simulink model "ap_12BAdapted"  (R2019b)
settings: Solver=FixedStepDiscrete  StartTime=0.0  StopTime=500  FixedStep=Ts  RelTol=1e-3  EnableMultiTasking=on
undefined symbols (not defined in the file): beaver_b, beaver_c, beaver_mass, beaver_S, Cl0, Cl_alpha2_dpt, Cl_beta, Cl_da, Cl_da_alpha, Cl_dr, Cl_p, Cl_r, Cm0, Cm_alpha, Cm_alpha2, Cm_beta2, Cm_de, Cm_df, Cm_dpt, Cm_q, Cm_r, Cn0, Cn_beta, Cn_beta3, Cn_da, Cn_dpt3, Cn_dr, Cn_p, Cn_q, Cn_r, Cx0, Cx_alpha, Cx_alpha2, Cx_alpha3, Cx_df, Cx_df_alpha, Cx_dpt, Cx_dpt2_alpha, Cx_dr, Cx_q, Cy0, Cy_beta, Cy_da, Cy_dr, Cy_dr_alpha, Cy_p, Cy_r, Cz0, Cz_alpha, Cz_alpha3, Cz_de, Cz_de_beta, Cz_df, Cz_df_alpha, Cz_dpt, Cz_q, d2r, fin_act_1, fin_act_2, fin_act_3 ... (+23)
libraries: simulink x10
(part 3 of 3)

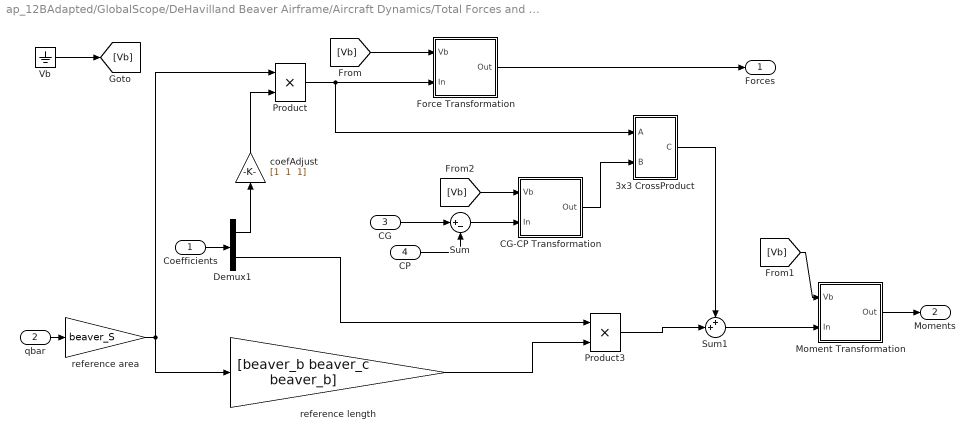
== system ap_12BAdapted/GlobalScope/DeHavilland Beaver Airframe/Aircraft Dynamics/Total Forces and Moments/Forces and Moments/Aero F&M ==
  Coefficients : Inport
  qbar : Inport  Port=2
  CG : Inport  Port=3
  CP : Inport  Port=4
  3x3 CrossProduct : Subsystem
  CG-CP Transformation : Subsystem  mask(Passive){}
      mask init:
      | %aeroicon('aeroblk');
  Demux1 : Demux  Outputs=[3,3]
  Force Transformation : Subsystem  mask(Passive){}
      mask init:
      | %aeroicon('aeroblk');
  Moment Transformation : Subsystem  mask(Passive){}
      mask init:
      | %aeroicon('aeroblk');
  Product : Product  SaturateOnIntegerOverflow=on  InputSameDT=on  OutDataTypeStr=Inherit: Same as first input
  Product3 : Product  SaturateOnIntegerOverflow=on  InputSameDT=on  OutDataTypeStr=Inherit: Same as first input
  Sum : Sum  Inputs=|+-  SaturateOnIntegerOverflow=on
  Sum1 : Sum  Inputs=++|  SaturateOnIntegerOverflow=on  InputSameDT=on  OutDataTypeStr=Inherit: Same as first input
  Vb : Ground
  coefAdjust : Gain  Gain="[1  1  1]"
  reference area : Gain  Gain=beaver_S  SaturateOnIntegerOverflow=on  OutDataTypeStr=Inherit: Same as input  ParamDataTypeStr=Inherit: Same as input
  reference length : Gain  Gain=[beaver_b beaver_c beaver_b]  SaturateOnIntegerOverflow=on  OutDataTypeStr=Inherit: Same as input  ParamDataTypeStr=Inherit: Same as input
  Forces : Outport  VectorParamsAs1DForOutWhenUnconnected=off
  Moments : Outport  Port=2  VectorParamsAs1DForOutWhenUnconnected=off
  wires:
  [Vb] -> Force Transformation/1(Vb)
  CP/1 -> Sum/2
  reference length/1 -> Product3/2
  Demux1/2 -> Product3/1
  qbar/1 -> reference area/1
  coefAdjust/1 -> Product/2
  Force Transformation/1(Out) -> Forces/1
  Demux1/1 -> coefAdjust/1
  Coefficients/1 -> Demux1/1
  [Vb] -> Moment Transformation/1(Vb)
  [Vb] -> CG-CP Transformation/1(Vb)
  CG-CP Transformation/1(Out) -> 3x3 CrossProduct/2(B)
  Product3/1 -> Sum1/2
  Vb/1 -> [Vb]
  reference area/1 -> reference length/1, Product/1
  Moment Transformation/1(Out) -> Moments/1
  Product/1 -> 3x3 CrossProduct/1(A), Force Transformation/2(In)
  Sum/1 -> CG-CP Transformation/2(In)
  Sum1/1 -> Moment Transformation/2(In)
  3x3 CrossProduct/1(C) -> Sum1/1
  CG/1 -> Sum/1

== system ap_12BAdapted/GlobalScope/DeHavilland Beaver Airframe/Aircraft Dynamics/6DoF (Quaternion)/Calculate DCM & Euler Angles/Quaternions to Direction Cosine Matrix/A11 ==
  normal(q) : Inport
  Demux : Demux
  Product{,1..3} (4 alike) : Product  RndMeth=Zero
  Sum : Sum  Inputs=++--
  A11 : Outport  VectorParamsAs1DForOutWhenUnconnected=off
  wires:
  Sum/1 -> A11/1
  Demux/4 -> Product/2, Product/1
  Demux/3 -> Product1/2, Product1/1
  Demux/2 -> Product2/2, Product2/1
  Demux/1 -> Product3/2, Product3/1
  Product3/1 -> Sum/1
  Product2/1 -> Sum/2
  Product1/1 -> Sum/3
  Product/1 -> Sum/4
  normal(q)/1 -> Demux/1

== system ap_12BAdapted/GlobalScope/DeHavilland Beaver Airframe/Aircraft Dynamics/6DoF (Quaternion)/Calculate DCM & Euler Angles/Quaternions to Direction Cosine Matrix/A12 ==
  normal(q) : Inport
  Demux : Demux
  Gain : Gain  Gain=2
  Product2 : Product  RndMeth=Zero
  Product3 : Product  RndMeth=Zero
  Sum : Sum  Inputs=|++
  A12 : Outport  VectorParamsAs1DForOutWhenUnconnected=off
  wires:
  Product2/1 -> Sum/2
  Product3/1 -> Sum/1
  Sum/1 -> Gain/1
  Demux/1 -> Product3/2
  Demux/2 -> Product2/1
  Demux/4 -> Product3/1
  Demux/3 -> Product2/2
  normal(q)/1 -> Demux/1
  Gain/1 -> A12/1

== system ap_12BAdapted/GlobalScope/DeHavilland Beaver Airframe/Aircraft Dynamics/6DoF (Quaternion)/Calculate DCM & Euler Angles/Quaternions to Direction Cosine Matrix/A13 ==
  normal(q) : Inport
  Demux : Demux
  Gain : Gain  Gain=2
  Product1 : Product  RndMeth=Zero
  Product2 : Product  RndMeth=Zero
  Sum : Sum  Inputs=|-+
  A13 : Outport  VectorParamsAs1DForOutWhenUnconnected=off
  wires:
  Demux/1 -> Product1/1
  Product1/1 -> Sum/1
  Product2/1 -> Sum/2
  Demux/4 -> Product2/2
  Demux/2 -> Product2/1
  Demux/3 -> Product1/2
  normal(q)/1 -> Demux/1
  Gain/1 -> A13/1
  Sum/1 -> Gain/1

== system ap_12BAdapted/GlobalScope/DeHavilland Beaver Airframe/Aircraft Dynamics/6DoF (Quaternion)/Calculate DCM & Euler Angles/Quaternions to Direction Cosine Matrix/A21 ==
  normal(q) : Inport
  Demux : Demux
  Gain : Gain  Gain=2
  Product2 : Product  RndMeth=Zero
  Product3 : Product  RndMeth=Zero
  Sum : Sum  Inputs=|-+
  A21 : Outport  VectorParamsAs1DForOutWhenUnconnected=off
  wires:
  Gain/1 -> A21/1
  normal(q)/1 -> Demux/1
  Demux/3 -> Product2/2
  Demux/4 -> Product3/1
  Demux/2 -> Product2/1
  Demux/1 -> Product3/2
  Sum/1 -> Gain/1
  Product3/1 -> Sum/1
  Product2/1 -> Sum/2

== system ap_12BAdapted/GlobalScope/DeHavilland Beaver Airframe/Aircraft Dynamics/6DoF (Quaternion)/Calculate DCM & Euler Angles/Quaternions to Direction Cosine Matrix/A22 ==
  normal(q) : Inport
  Demux : Demux
  Product{,1..3} (4 alike) : Product  RndMeth=Zero
  Sum : Sum  Inputs=+-+-
  A22 : Outport  VectorParamsAs1DForOutWhenUnconnected=off
  wires:
  normal(q)/1 -> Demux/1
  Product/1 -> Sum/4
  Product1/1 -> Sum/3
  Product2/1 -> Sum/2
  Product3/1 -> Sum/1
  Demux/1 -> Product3/1, Product3/2
  Demux/2 -> Product2/1, Product2/2
  Demux/3 -> Product1/1, Product1/2
  Demux/4 -> Product/1, Product/2
  Sum/1 -> A22/1

== system ap_12BAdapted/GlobalScope/DeHavilland Beaver Airframe/Aircraft Dynamics/6DoF (Quaternion)/Calculate DCM & Euler Angles/Quaternions to Direction Cosine Matrix/A23 ==
  normal(q) : Inport
  Demux : Demux
  Gain : Gain  Gain=2
  Product1 : Product  RndMeth=Zero
  Product2 : Product  RndMeth=Zero
  Sum : Sum  Inputs=|++
  A23 : Outport  VectorParamsAs1DForOutWhenUnconnected=off
  wires:
  Demux/4 -> Product2/2
  Product2/1 -> Sum/2
  Product1/1 -> Sum/1
  Sum/1 -> Gain/1
  Demux/1 -> Product1/1
  Demux/2 -> Product1/2
  Demux/3 -> Product2/1
  Gain/1 -> A23/1
  normal(q)/1 -> Demux/1

== system ap_12BAdapted/GlobalScope/DeHavilland Beaver Airframe/Aircraft Dynamics/6DoF (Quaternion)/Calculate DCM & Euler Angles/Quaternions to Direction Cosine Matrix/A31 ==
  normal(q) : Inport
  Demux : Demux
  Gain : Gain  Gain=2
  Product1 : Product  RndMeth=Zero
  Product2 : Product  RndMeth=Zero
  Sum : Sum  Inputs=|++
  A31 : Outport  VectorParamsAs1DForOutWhenUnconnected=off
  wires:
  Sum/1 -> Gain/1
  Gain/1 -> A31/1
  normal(q)/1 -> Demux/1
  Demux/3 -> Product1/2
  Demux/2 -> Product2/1
  Demux/4 -> Product2/2
  Product2/1 -> Sum/2
  Product1/1 -> Sum/1
  Demux/1 -> Product1/1

== system ap_12BAdapted/GlobalScope/DeHavilland Beaver Airframe/Aircraft Dynamics/6DoF (Quaternion)/Calculate DCM & Euler Angles/Quaternions to Direction Cosine Matrix/A32 ==
  normal(q) : Inport
  Demux : Demux
  Gain : Gain  Gain=2
  Product1 : Product  RndMeth=Zero
  Product2 : Product  RndMeth=Zero
  Sum : Sum  Inputs=|-+
  A32 : Outport  VectorParamsAs1DForOutWhenUnconnected=off
  wires:
  normal(q)/1 -> Demux/1
  Gain/1 -> A32/1
  Demux/3 -> Product2/1
  Demux/2 -> Product1/2
  Demux/1 -> Product1/1
  Sum/1 -> Gain/1
  Product1/1 -> Sum/1
  Product2/1 -> Sum/2
  Demux/4 -> Product2/2

== system ap_12BAdapted/GlobalScope/DeHavilland Beaver Airframe/Aircraft Dynamics/6DoF (Quaternion)/Calculate DCM & Euler Angles/Quaternions to Direction Cosine Matrix/A33 ==
  normal(q) : Inport
  Demux : Demux
  Product{,1..3} (4 alike) : Product  RndMeth=Zero
  Sum : Sum  Inputs=+--+
  A33 : Outport  VectorParamsAs1DForOutWhenUnconnected=off
  wires:
  normal(q)/1 -> Demux/1
  Product/1 -> Sum/4
  Product1/1 -> Sum/3
  Product2/1 -> Sum/2
  Product3/1 -> Sum/1
  Demux/1 -> Product3/1, Product3/2
  Demux/2 -> Product2/1, Product2/2
  Demux/3 -> Product1/1, Product1/2
  Demux/4 -> Product/1, Product/2
  Sum/1 -> A33/1

== system ap_12BAdapted/GlobalScope/DeHavilland Beaver Airframe/Aircraft Dynamics/6DoF (Quaternion)/Calculate DCM & Euler Angles/Quaternions to Direction Cosine Matrix/Create 3x3 Matrix ==
  M11 : Inport  PortDimensions=1
  M12 : Inport  Port=2  PortDimensions=1
  M13 : Inport  Port=3  PortDimensions=1
  M21 : Inport  Port=4  PortDimensions=1
  M22 : Inport  Port=5  PortDimensions=1
  M23 : Inport  Port=6  PortDimensions=1
  M31 : Inport  Port=7  PortDimensions=1
  M32 : Inport  Port=8  PortDimensions=1
  M33 : Inport  Port=9  PortDimensions=1
  Reshape (9) to [3x3] column-major : Reshape  OutputDimensionality=Customize  OutputDimensions=[3,3]
  Vector Concatenate : Concatenate  NumInputs=9
  Matrix : Outport  PortDimensions=[3 3]  VectorParamsAs1DForOutWhenUnconnected=off
  wires:
  M33/1 -> Vector Concatenate/9
  M23/1 -> Vector Concatenate/8
  M13/1 -> Vector Concatenate/7
  M32/1 -> Vector Concatenate/6
  Reshape (9) to [3x3] column-major/1 -> Matrix/1
  M22/1 -> Vector Concatenate/5
  M12/1 -> Vector Concatenate/4
  M31/1 -> Vector Concatenate/3
  M21/1 -> Vector Concatenate/2
  M11/1 -> Vector Concatenate/1
  Vector Concatenate/1 -> Reshape (9) to [3x3] column-major/1

== system ap_12BAdapted/GlobalScope/DeHavilland Beaver Airframe/Aircraft Dynamics/6DoF (Quaternion)/Calculate DCM & Euler Angles/Quaternions to Direction Cosine Matrix/Quaternion Normalize ==
  q : Inport  Unit=1
  Demux : Demux
  Mux : Mux
  Product{,1..3} (4 alike) : Product  Inputs=*/
  Quaternion Modulus : Subsystem  mask(Quaternion Modulus){}
      mask help: shared_aeroblks:sharedaeroblkutil:blockQuaternionModulusDesc
      mask init:
      | if license('test','aerospace_blockset')
      |     aerosharedicon('shared');
      | elseif license('test','powertrain_blockset')
      |     sharedautoicon('shared');
      | end
      mask Help: eval('if license(''test'',''aerospace_blockset'')aerosharedhelp;elseif license(''test'',''powertrain_blockset'')sharedautohelp;end')
  normal(q) : Outport  Unit=1  VectorParamsAs1DForOutWhenUnconnected=off
  wires:
  Product3/1 -> Mux/4
  Product2/1 -> Mux/3
  Product1/1 -> Mux/2
  Product/1 -> Mux/1
  Quaternion Modulus/1(|q|) -> Product3/2, Product2/2, Product/2, Product1/2
  q/1 -> Demux/1, Quaternion Modulus/1(q)
  Mux/1 -> normal(q)/1
  Demux/1 -> Product/1
  Demux/2 -> Product1/1
  Demux/3 -> Product2/1
  Demux/4 -> Product3/1

== system ap_12BAdapted/GlobalScope/DeHavilland Beaver Airframe/Aircraft Dynamics/6DoF (Quaternion)/Calculate DCM & Euler Angles/Quaternions to Rotation Angles (ZYX)/Quaternion Normalize ==
  q : Inport
  Demux : Demux
  Mux : Mux
  Product{,1..3} (4 alike) : Product  Inputs=*/
  Quaternion Modulus : Subsystem
  normal(q) : Outport  VectorParamsAs1DForOutWhenUnconnected=off
  wires:
  Product3/1 -> Mux/4
  Product1/1 -> Mux/2
  Demux/1 -> Product/1
  Quaternion Modulus/1(|q|) -> Product1/2, Product/2, Product2/2, Product3/2
  Mux/1 -> normal(q)/1
  q/1 -> Quaternion Modulus/1(q), Demux/1
  Product/1 -> Mux/1
  Demux/3 -> Product2/1
  Demux/4 -> Product3/1
  Product2/1 -> Mux/3
  Demux/2 -> Product1/1

== system ap_12BAdapted/GlobalScope/DeHavilland Beaver Airframe/Aircraft Dynamics/6DoF (Quaternion)/Calculate omega_dot/3x3 CrossProduct/Subsystem ==
  A : Inport
  B : Inport  Port=2
  Demux : Demux  Outputs=3
  Demux1 : Demux  Outputs=3
  Mux : Mux  Inputs=3
  i x j : Product  SaturateOnIntegerOverflow=on  InputSameDT=on  OutDataTypeStr=Inherit: Same as first input
  j x k : Product  SaturateOnIntegerOverflow=on  InputSameDT=on  OutDataTypeStr=Inherit: Same as first input
  k x i : Product  SaturateOnIntegerOverflow=on  InputSameDT=on  OutDataTypeStr=Inherit: Same as first input
  Out1 : Outport  VectorParamsAs1DForOutWhenUnconnected=off
  wires:
  Demux1/3 -> j x k/2
  Demux/2 -> j x k/1
  Demux/3 -> k x i/1
  Demux1/1 -> k x i/2
  Demux1/2 -> i x j/2
  Demux/1 -> i x j/1
  i x j/1 -> Mux/3
  k x i/1 -> Mux/2
  j x k/1 -> Mux/1
  B/1 -> Demux1/1
  A/1 -> Demux/1
  Mux/1 -> Out1/1

== system ap_12BAdapted/GlobalScope/DeHavilland Beaver Airframe/Aircraft Dynamics/6DoF (Quaternion)/Calculate omega_dot/3x3 CrossProduct/Subsystem1 ==
  A : Inport
  B : Inport  Port=2
  Demux : Demux  Outputs=3
  Demux1 : Demux  Outputs=3
  Mux : Mux  Inputs=3
  i x k : Product  SaturateOnIntegerOverflow=on  InputSameDT=on  OutDataTypeStr=Inherit: Same as first input
  j x i : Product  SaturateOnIntegerOverflow=on  InputSameDT=on  OutDataTypeStr=Inherit: Same as first input
  k x j : Product  SaturateOnIntegerOverflow=on  InputSameDT=on  OutDataTypeStr=Inherit: Same as first input
  Out1 : Outport  VectorParamsAs1DForOutWhenUnconnected=off
  wires:
  j x i/1 -> Mux/3
  i x k/1 -> Mux/2
  k x j/1 -> Mux/1
  Mux/1 -> Out1/1
  Demux1/1 -> j x i/2
  Demux/2 -> j x i/1
  Demux1/3 -> i x k/2
  Demux/1 -> i x k/1
  Demux1/2 -> k x j/2
  Demux/3 -> k x j/1
  B/1 -> Demux1/1
  A/1 -> Demux/1

== system ap_12BAdapted/GlobalScope/DeHavilland Beaver Airframe/Aircraft Dynamics/Total Forces and Moments/Actuators/sof/ResetIntegratorInternal ==
  note: ic
  note: Level Reset Integration With Saturation
      | y(n) = y(n-1) + K*Ts*u(n-1)
  U : Inport
  R : Inport  Port=2
  ic : Inport  Port=3
  Constant : Constant  Value=1.0
  Constant1 : Constant  Value=Ts
  Product : Product  RndMeth=Zero
  Product1 : Product  RndMeth=Zero
  Sum3 : Sum
  Switch : Switch  Criteria=u2 ~= 0
  Switch1 : Switch  Criteria=u2 ~= 0
  X : UnitDelay  SampleTime=Ts  HasFrameUpgradeWarning=on
  Y : Outport  VectorParamsAs1DForOutWhenUnconnected=off
  wires:
  Product1/1 -> Sum3/1
  U/1 -> Product1/2
  Sum3/1 -> Switch1/3
  Product/1 -> Product1/1
  ic/1 -> Switch1/1, Switch/1
  Constant1/1 -> Product/2  "deltaT"
  Switch1/1 -> X/1
  Constant/1 -> Product/1  "gain"
  Switch/1 -> Y/1, Sum3/2
  R/1 -> Switch1/2, Switch/2
  X/1 -> Switch/3

== system ap_12BAdapted/GlobalScope/DeHavilland Beaver Airframe/Aircraft Dynamics/Total Forces and Moments/Actuators/sof/ResetIntegratorInternal1 ==
  note: Level Reset Integration With Saturation
      | y(n) = y(n-1) + K*Ts*u(n-1)
  note: ic
  U : Inport
  R : Inport  Port=2
  ic : Inport  Port=3
  Constant : Constant  Value=1.0
  Constant1 : Constant  Value=Ts
  Product : Product  RndMeth=Zero
  Product1 : Product  RndMeth=Zero
  Saturation : Saturate  UpperLimit=fin_max  LowerLimit=fin_min
  Sum3 : Sum
  Switch : Switch  Criteria=u2 ~= 0
  Switch1 : Switch  Criteria=u2 ~= 0
  X : UnitDelay  SampleTime=Ts  HasFrameUpgradeWarning=on
  Y : Outport  VectorParamsAs1DForOutWhenUnconnected=off
  wires:
  X/1 -> Switch/3
  R/1 -> Switch/2, Switch1/2
  Saturation/1 -> Sum3/2, Y/1
  Constant/1 -> Product/1  "gain"
  Switch1/1 -> X/1
  Constant1/1 -> Product/2  "deltaT"
  ic/1 -> Switch/1, Switch1/1
  Switch/1 -> Saturation/1
  Product/1 -> Product1/1
  Sum3/1 -> Switch1/3
  U/1 -> Product1/2
  Product1/1 -> Sum3/1

== system ap_12BAdapted/GlobalScope/DeHavilland Beaver Airframe/Aircraft Dynamics/Total Forces and Moments/Actuators/sof/ic1 ==
  Constant : Constant  Value=0
  Constant1 : Constant  Value=fin_act_1
  Unit Delay : UnitDelay  InitialCondition=1  SampleTime=-1  HasFrameUpgradeWarning=on
  R : Outport  VectorParamsAs1DForOutWhenUnconnected=off
  IC : Outport  Port=2  VectorParamsAs1DForOutWhenUnconnected=off
  wires:
  Constant1/1 -> IC/1
  Unit Delay/1 -> R/1
  Constant/1 -> Unit Delay/1

== system ap_12BAdapted/GlobalScope/DeHavilland Beaver Airframe/Aircraft Dynamics/Total Forces and Moments/Actuators/sof/ic3 ==
  Constant : Constant  Value=0
  Constant1 : Constant  Value=0.0
  Unit Delay : UnitDelay  InitialCondition=1  SampleTime=-1  HasFrameUpgradeWarning=on
  R : Outport  VectorParamsAs1DForOutWhenUnconnected=off
  IC : Outport  Port=2  VectorParamsAs1DForOutWhenUnconnected=off
  wires:
  Constant/1 -> Unit Delay/1
  Unit Delay/1 -> R/1
  Constant1/1 -> IC/1

== system ap_12BAdapted/GlobalScope/DeHavilland Beaver Airframe/Aircraft Dynamics/Total Forces and Moments/Actuators/sof1/ResetIntegratorInternal ==
  note: Level Reset Integration With Saturation
      | y(n) = y(n-1) + K*Ts*u(n-1)
  note: ic
  U : Inport
  R : Inport  Port=2
  ic : Inport  Port=3
  Constant : Constant  Value=1.0
  Constant1 : Constant  Value=Ts
  Product : Product  RndMeth=Zero
  Product1 : Product  RndMeth=Zero
  Sum3 : Sum
  Switch : Switch  Criteria=u2 ~= 0
  Switch1 : Switch  Criteria=u2 ~= 0
  X : UnitDelay  SampleTime=Ts  HasFrameUpgradeWarning=on
  Y : Outport  VectorParamsAs1DForOutWhenUnconnected=off
  wires:
  X/1 -> Switch/3
  R/1 -> Switch/2, Switch1/2
  Switch/1 -> Sum3/2, Y/1
  Constant/1 -> Product/1  "gain"
  Switch1/1 -> X/1
  Constant1/1 -> Product/2  "deltaT"
  ic/1 -> Switch/1, Switch1/1
  Product/1 -> Product1/1
  Sum3/1 -> Switch1/3
  U/1 -> Product1/2
  Product1/1 -> Sum3/1

== system ap_12BAdapted/GlobalScope/DeHavilland Beaver Airframe/Aircraft Dynamics/Total Forces and Moments/Actuators/sof1/ResetIntegratorInternal1 ==
  note: ic
  note: Level Reset Integration With Saturation
      | y(n) = y(n-1) + K*Ts*u(n-1)
  U : Inport
  R : Inport  Port=2
  ic : Inport  Port=3
  Constant : Constant  Value=1.0
  Constant1 : Constant  Value=Ts
  Product : Product  RndMeth=Zero
  Product1 : Product  RndMeth=Zero
  Saturation : Saturate  UpperLimit=fin_max  LowerLimit=fin_min
  Sum3 : Sum
  Switch : Switch  Criteria=u2 ~= 0
  Switch1 : Switch  Criteria=u2 ~= 0
  X : UnitDelay  SampleTime=Ts  HasFrameUpgradeWarning=on
  Y : Outport  VectorParamsAs1DForOutWhenUnconnected=off
  wires:
  Product1/1 -> Sum3/1
  U/1 -> Product1/2
  Sum3/1 -> Switch1/3
  Product/1 -> Product1/1
  Switch/1 -> Saturation/1
  ic/1 -> Switch1/1, Switch/1
  Constant1/1 -> Product/2  "deltaT"
  Switch1/1 -> X/1
  Constant/1 -> Product/1  "gain"
  Saturation/1 -> Y/1, Sum3/2
  R/1 -> Switch1/2, Switch/2
  X/1 -> Switch/3

== system ap_12BAdapted/GlobalScope/DeHavilland Beaver Airframe/Aircraft Dynamics/Total Forces and Moments/Actuators/sof1/ic1 ==
  Constant : Constant  Value=0
  Constant1 : Constant  Value=fin_act_2
  Unit Delay : UnitDelay  InitialCondition=1  SampleTime=-1  HasFrameUpgradeWarning=on
  R : Outport  VectorParamsAs1DForOutWhenUnconnected=off
  IC : Outport  Port=2  VectorParamsAs1DForOutWhenUnconnected=off
  wires:
  Constant/1 -> Unit Delay/1
  Unit Delay/1 -> R/1
  Constant1/1 -> IC/1

== system ap_12BAdapted/GlobalScope/DeHavilland Beaver Airframe/Aircraft Dynamics/Total Forces and Moments/Actuators/sof1/ic3 ==
  Constant : Constant  Value=0
  Constant1 : Constant  Value=0.0
  Unit Delay : UnitDelay  InitialCondition=1  SampleTime=-1  HasFrameUpgradeWarning=on
  R : Outport  VectorParamsAs1DForOutWhenUnconnected=off
  IC : Outport  Port=2  VectorParamsAs1DForOutWhenUnconnected=off
  wires:
  Constant1/1 -> IC/1
  Unit Delay/1 -> R/1
  Constant/1 -> Unit Delay/1

== system ap_12BAdapted/GlobalScope/DeHavilland Beaver Airframe/Aircraft Dynamics/Total Forces and Moments/Actuators/sof2/ResetIntegratorInternal ==
  note: ic
  note: Level Reset Integration With Saturation
      | y(n) = y(n-1) + K*Ts*u(n-1)
  U : Inport
  R : Inport  Port=2
  ic : Inport  Port=3
  Constant : Constant  Value=1.0
  Constant1 : Constant  Value=Ts
  Product : Product  RndMeth=Zero
  Product1 : Product  RndMeth=Zero
  Sum3 : Sum
  Switch : Switch  Criteria=u2 ~= 0
  Switch1 : Switch  Criteria=u2 ~= 0
  X : UnitDelay  SampleTime=Ts  HasFrameUpgradeWarning=on
  Y : Outport  VectorParamsAs1DForOutWhenUnconnected=off
  wires:
  Product1/1 -> Sum3/1
  U/1 -> Product1/2
  Sum3/1 -> Switch1/3
  Product/1 -> Product1/1
  ic/1 -> Switch1/1, Switch/1
  Constant1/1 -> Product/2  "deltaT"
  Switch1/1 -> X/1
  Constant/1 -> Product/1  "gain"
  Switch/1 -> Y/1, Sum3/2
  R/1 -> Switch1/2, Switch/2
  X/1 -> Switch/3

== system ap_12BAdapted/GlobalScope/DeHavilland Beaver Airframe/Aircraft Dynamics/Total Forces and Moments/Actuators/sof2/ResetIntegratorInternal1 ==
  note: Level Reset Integration With Saturation
      | y(n) = y(n-1) + K*Ts*u(n-1)
  note: ic
  U : Inport
  R : Inport  Port=2
  ic : Inport  Port=3
  Constant : Constant  Value=1.0
  Constant1 : Constant  Value=Ts
  Product : Product  RndMeth=Zero
  Product1 : Product  RndMeth=Zero
  Saturation : Saturate  UpperLimit=fin_max  LowerLimit=fin_min
  Sum3 : Sum
  Switch : Switch  Criteria=u2 ~= 0
  Switch1 : Switch  Criteria=u2 ~= 0
  X : UnitDelay  SampleTime=Ts  HasFrameUpgradeWarning=on
  Y : Outport  VectorParamsAs1DForOutWhenUnconnected=off
  wires:
  X/1 -> Switch/3
  R/1 -> Switch/2, Switch1/2
  Saturation/1 -> Sum3/2, Y/1
  Constant/1 -> Product/1  "gain"
  Switch1/1 -> X/1
  Constant1/1 -> Product/2  "deltaT"
  ic/1 -> Switch/1, Switch1/1
  Switch/1 -> Saturation/1
  Product/1 -> Product1/1
  Sum3/1 -> Switch1/3
  U/1 -> Product1/2
  Product1/1 -> Sum3/1

== system ap_12BAdapted/GlobalScope/DeHavilland Beaver Airframe/Aircraft Dynamics/Total Forces and Moments/Actuators/sof2/ic1 ==
  Constant : Constant  Value=0
  Constant1 : Constant  Value=fin_act_3
  Unit Delay : UnitDelay  InitialCondition=1  SampleTime=-1  HasFrameUpgradeWarning=on
  R : Outport  VectorParamsAs1DForOutWhenUnconnected=off
  IC : Outport  Port=2  VectorParamsAs1DForOutWhenUnconnected=off
  wires:
  Constant1/1 -> IC/1
  Unit Delay/1 -> R/1
  Constant/1 -> Unit Delay/1

== system ap_12BAdapted/GlobalScope/DeHavilland Beaver Airframe/Aircraft Dynamics/Total Forces and Moments/Actuators/sof2/ic3 ==
  Constant : Constant  Value=0
  Constant1 : Constant  Value=0.0
  Unit Delay : UnitDelay  InitialCondition=1  SampleTime=-1  HasFrameUpgradeWarning=on
  R : Outport  VectorParamsAs1DForOutWhenUnconnected=off
  IC : Outport  Port=2  VectorParamsAs1DForOutWhenUnconnected=off
  wires:
  Constant/1 -> Unit Delay/1
  Unit Delay/1 -> R/1
  Constant1/1 -> IC/1

== system ap_12BAdapted/GlobalScope/DeHavilland Beaver Airframe/Aircraft Dynamics/Total Forces and Moments/Aerodynamics/Actuator Increments/Aileron ==
  alpha : Inport
  Actuators : Inport  Port=2
  Gain1 : Gain  Gain=0  SaturateOnIntegerOverflow=on  OutDataTypeStr=Inherit: Same as input  ParamDataTypeStr=Inherit: Same as input
  Gain2 : Gain  Gain=Cy_da  SaturateOnIntegerOverflow=on  OutDataTypeStr=Inherit: Same as input  ParamDataTypeStr=Inherit: Same as input
  Gain3 : Gain  Gain=0  SaturateOnIntegerOverflow=on  OutDataTypeStr=Inherit: Same as input  ParamDataTypeStr=Inherit: Same as input
  Gain4 : Gain  Gain=Cn_da  SaturateOnIntegerOverflow=on  OutDataTypeStr=Inherit: Same as input  ParamDataTypeStr=Inherit: Same as input
  Gain5 : Gain  Gain=0  SaturateOnIntegerOverflow=on  OutDataTypeStr=Inherit: Same as input  ParamDataTypeStr=Inherit: Same as input
  Gain6 : Gain  Gain=Cl_da  SaturateOnIntegerOverflow=on  OutDataTypeStr=Inherit: Same as input  ParamDataTypeStr=Inherit: Same as input
  Gain7 : Gain  Gain=Cl_da_alpha  SaturateOnIntegerOverflow=on  OutDataTypeStr=Inherit: Same as input  ParamDataTypeStr=Inherit: Same as input
  Mux1 : Mux  Inputs=6
  Product4 : Product  SaturateOnIntegerOverflow=on  InputSameDT=on  OutDataTypeStr=Inherit: Same as first input
  Selector1 : Selector  InputPortWidth=4  IndexOptions=Index vector (dialog)  Indices=2  OutputSizes=1
  Sum1 : Sum  Inputs=++|  SaturateOnIntegerOverflow=on
  delCoeff : Outport  VectorParamsAs1DForOutWhenUnconnected=off
  wires:
  Gain6/1 -> Sum1/1
  Sum1/1 -> Mux1/4
  Gain7/1 -> Sum1/2
  Product4/1 -> Gain7/1
  Gain1/1 -> Mux1/1  "Cx"
  alpha/1 -> Product4/2
  Actuators/1 -> Selector1/1
  Mux1/1 -> delCoeff/1
  Gain2/1 -> Mux1/2  "Cy"
  Gain3/1 -> Mux1/3  "Cz"
  Gain5/1 -> Mux1/5  "Cm"
  Gain4/1 -> Mux1/6
  Selector1/1 -> Gain1/1, Gain2/1, Gain3/1, Gain6/1, Product4/1, Gain5/1, Gain4/1

== system ap_12BAdapted/GlobalScope/DeHavilland Beaver Airframe/Aircraft Dynamics/Total Forces and Moments/Aerodynamics/Actuator Increments/Elevator ==
  Actuators : Inport
  Beta : Inport  Port=2
  Constant1 : Constant  Value=0
  Gain1 : Gain  Gain=Cz_de  SaturateOnIntegerOverflow=on  OutDataTypeStr=Inherit: Same as input  ParamDataTypeStr=Inherit: Same as input
  Gain2 : Gain  Gain=Cz_de_beta  SaturateOnIntegerOverflow=on  OutDataTypeStr=Inherit: Same as input  ParamDataTypeStr=Inherit: Same as input
  Gain3 : Gain  Gain=Cm_de  SaturateOnIntegerOverflow=on  OutDataTypeStr=Inherit: Same as input  ParamDataTypeStr=Inherit: Same as input
  Mux1 : Mux  Inputs=6
  Product1 : Product  SaturateOnIntegerOverflow=on  InputSameDT=on  OutDataTypeStr=Inherit: Same as first input
  Product2 : Product  SaturateOnIntegerOverflow=on  InputSameDT=on  OutDataTypeStr=Inherit: Same as first input
  Selector1 : Selector  InputPortWidth=4  IndexOptions=Index vector (dialog)  Indices=1  OutputSizes=1
  Sum1 : Sum  SaturateOnIntegerOverflow=on
  delCoeff : Outport  VectorParamsAs1DForOutWhenUnconnected=off
  wires:
  Gain3/1 -> Mux1/5
  Gain1/1 -> Sum1/2
  Gain2/1 -> Sum1/1
  Sum1/1 -> Mux1/3
  Product2/1 -> Gain2/1
  Beta/1 -> Product1/2, Product1/1
  Mux1/1 -> delCoeff/1
  Selector1/1 -> Gain3/1, Product2/2, Gain1/1
  Constant1/1 -> Mux1/1, Mux1/2, Mux1/4, Mux1/6
  Actuators/1 -> Selector1/1
  Product1/1 -> Product2/1

== system ap_12BAdapted/GlobalScope/DeHavilland Beaver Airframe/Aircraft Dynamics/Total Forces and Moments/Aerodynamics/Actuator Increments/Flap ==
  Alpha : Inport
  Actuators : Inport  Port=2
  Constant1 : Constant  Value=0
  Constant2 : Constant  Value=0
  Constant3 : Constant  Value=0
  Gain1 : Gain  Gain=Cx_df  SaturateOnIntegerOverflow=on  OutDataTypeStr=Inherit: Same as input  ParamDataTypeStr=Inherit: Same as input
  Gain2 : Gain  Gain=Cx_df_alpha  SaturateOnIntegerOverflow=on  OutDataTypeStr=Inherit: Same as input  ParamDataTypeStr=Inherit: Same as input
  Gain3 : Gain  Gain=Cz_df  SaturateOnIntegerOverflow=on  OutDataTypeStr=Inherit: Same as input  ParamDataTypeStr=Inherit: Same as input
  Gain4 : Gain  Gain=Cz_df_alpha  SaturateOnIntegerOverflow=on  OutDataTypeStr=Inherit: Same as input  ParamDataTypeStr=Inherit: Same as input
  Gain5 : Gain  Gain=Cm_df  SaturateOnIntegerOverflow=on  OutDataTypeStr=Inherit: Same as input  ParamDataTypeStr=Inherit: Same as input
  Mux1 : Mux  Inputs=6
  Product1 : Product  SaturateOnIntegerOverflow=on  InputSameDT=on  OutDataTypeStr=Inherit: Same as first input
  Product4 : Product  SaturateOnIntegerOverflow=on  InputSameDT=on  OutDataTypeStr=Inherit: Same as first input
  Selector1 : Selector  InputPortWidth=4  IndexOptions=Index vector (dialog)  Indices=4  OutputSizes=1
  Sum1 : Sum  SaturateOnIntegerOverflow=on
  Sum2 : Sum  SaturateOnIntegerOverflow=on
  delCoeff : Outport  VectorParamsAs1DForOutWhenUnconnected=off
  wires:
  Selector1/1 -> Gain1/1, Product4/1, Product1/1, Gain3/1, Gain5/1
  Actuators/1 -> Selector1/1
  Gain5/1 -> Mux1/5
  Gain3/1 -> Sum2/1
  Gain4/1 -> Sum2/2
  Product1/1 -> Gain4/1
  Gain1/1 -> Sum1/1
  Gain2/1 -> Sum1/2
  Product4/1 -> Gain2/1
  Alpha/1 -> Product1/2, Product4/2
  Mux1/1 -> delCoeff/1
  Sum1/1 -> Mux1/1
  Sum2/1 -> Mux1/3
  Constant1/1 -> Mux1/2
  Constant2/1 -> Mux1/4
  Constant3/1 -> Mux1/6

== system ap_12BAdapted/GlobalScope/DeHavilland Beaver Airframe/Aircraft Dynamics/Total Forces and Moments/Aerodynamics/Actuator Increments/Rudder ==
  Alpha : Inport
  Actuators : Inport  Port=2
  Constant1 : Constant  Value=0
  Constant2 : Constant  Value=0
  Gain1 : Gain  Gain=Cl_dr  SaturateOnIntegerOverflow=on  OutDataTypeStr=Inherit: Same as input  ParamDataTypeStr=Inherit: Same as input
  Gain2 : Gain  Gain=Cn_dr  SaturateOnIntegerOverflow=on  OutDataTypeStr=Inherit: Same as input  ParamDataTypeStr=Inherit: Same as input
  Gain3 : Gain  Gain=Cy_dr_alpha  SaturateOnIntegerOverflow=on  OutDataTypeStr=Inherit: Same as input  ParamDataTypeStr=Inherit: Same as input
  Gain4 : Gain  Gain=Cy_dr  SaturateOnIntegerOverflow=on  OutDataTypeStr=Inherit: Same as input  ParamDataTypeStr=Inherit: Same as input
  Gain5 : Gain  Gain=Cx_dr  SaturateOnIntegerOverflow=on  OutDataTypeStr=Inherit: Same as input  ParamDataTypeStr=Inherit: Same as input
  Mux1 : Mux  Inputs=6
  Product1 : Product  SaturateOnIntegerOverflow=on  InputSameDT=on  OutDataTypeStr=Inherit: Same as first input
  Selector1 : Selector  InputPortWidth=4  IndexOptions=Index vector (dialog)  Indices=3  OutputSizes=1
  Sum1 : Sum  SaturateOnIntegerOverflow=on
  delCoeff : Outport  VectorParamsAs1DForOutWhenUnconnected=off
  wires:
  Gain5/1 -> Mux1/1
  Gain4/1 -> Sum1/1
  Gain3/1 -> Sum1/2
  Gain1/1 -> Mux1/4
  Gain2/1 -> Mux1/6
  Product1/1 -> Gain3/1
  Alpha/1 -> Product1/2
  Mux1/1 -> delCoeff/1
  Actuators/1 -> Selector1/1
  Sum1/1 -> Mux1/2
  Constant1/1 -> Mux1/3
  Constant2/1 -> Mux1/5
  Selector1/1 -> Gain5/1, Gain4/1, Product1/1, Gain1/1, Gain2/1

== system ap_12BAdapted/GlobalScope/DeHavilland Beaver Airframe/Aircraft Dynamics/Total Forces and Moments/Aerodynamics/Body Rate Damping/p ==
  Constant1 : Constant  Value=0
  Constant2 : Constant  Value=Cy_p
  Constant3 : Constant  Value=Cl_p
  Constant4 : Constant  Value=Cn_p
  Mux1 : Mux  Inputs=6
  delCoeff : Outport  VectorParamsAs1DForOutWhenUnconnected=off
  wires:
  Constant2/1 -> Mux1/2
  Mux1/1 -> delCoeff/1
  Constant1/1 -> Mux1/5, Mux1/3, Mux1/1
  Constant4/1 -> Mux1/6
  Constant3/1 -> Mux1/4

== system ap_12BAdapted/GlobalScope/DeHavilland Beaver Airframe/Aircraft Dynamics/Total Forces and Moments/Aerodynamics/Body Rate Damping/q ==
  Constant1 : Constant  Value=0
  Constant2 : Constant  Value=Cz_q
  Constant3 : Constant  Value=Cx_q
  Constant4 : Constant  Value=Cm_q
  Constant5 : Constant  Value=Cn_q
  Mux1 : Mux  Inputs=6
  delCoeff : Outport  VectorParamsAs1DForOutWhenUnconnected=off
  wires:
  Constant2/1 -> Mux1/3
  Constant5/1 -> Mux1/6
  Constant1/1 -> Mux1/4, Mux1/2
  Constant4/1 -> Mux1/5
  Constant3/1 -> Mux1/1
  Mux1/1 -> delCoeff/1

== system ap_12BAdapted/GlobalScope/DeHavilland Beaver Airframe/Aircraft Dynamics/Total Forces and Moments/Aerodynamics/Body Rate Damping/r ==
  Constant : Constant  Value=0
  Constant1 : Constant  Value=Cy_r
  Constant2 : Constant  Value=Cl_r
  Constant3 : Constant  Value=Cm_r
  Constant4 : Constant  Value=Cn_r
  Mux1 : Mux  Inputs=6
  delCoeff : Outport  VectorParamsAs1DForOutWhenUnconnected=off
  wires:
  Constant3/1 -> Mux1/5
  Constant1/1 -> Mux1/2
  Constant4/1 -> Mux1/6
  Constant2/1 -> Mux1/4
  Constant/1 -> Mux1/3, Mux1/1
  Mux1/1 -> delCoeff/1

== system ap_12BAdapted/GlobalScope/DeHavilland Beaver Airframe/Aircraft Dynamics/Total Forces and Moments/Engine /pow/calc ==
  In1 : Inport
  Constant4 : Constant  Value=408.0
  Constant5 : Constant  Value=1.0
  Demux : Demux  Outputs=3
  Gain2 : Gain  Gain=0.0965  SaturateOnIntegerOverflow=on  OutDataTypeStr=Inherit: Same as input  ParamDataTypeStr=Inherit: Same as input
  Gain4 : Gain  Gain=0.8163  SaturateOnIntegerOverflow=on  OutDataTypeStr=Inherit: Same as input  ParamDataTypeStr=Inherit: Same as input
  Product2 : Product  RndMeth=Zero
  Sum1 : Sum  Inputs=+-|  SaturateOnIntegerOverflow=on
  Sum2 : Sum  Inputs=+-|  SaturateOnIntegerOverflow=on
  Terminator : Terminator
  Out1 : Outport  VectorParamsAs1DForOutWhenUnconnected=off
  wires:
  In1/1 -> Demux/1
  Product2/1 -> Out1/1
  Sum2/1 -> Product2/2
  Constant5/1 -> Sum2/1
  Gain4/1 -> Sum2/2
  Constant4/1 -> Sum1/1
  Demux/1 -> Gain2/1
  Demux/2 -> Terminator/1
  Gain2/1 -> Sum1/2
  Sum1/1 -> Product2/1
  Demux/3 -> Gain4/1

== system ap_12BAdapted/GlobalScope/DeHavilland Beaver Airframe/Aircraft Dynamics/Total Forces and Moments/Engine /pow/calc1 ==
  In1 : Inport
  Constant1 : Constant  Value=2010
  Constant2 : Constant  Value=7.4
  Demux : Demux  Outputs=2
  Product1 : Product  RndMeth=Zero
  Sum3 : Sum  Inputs=++|  SaturateOnIntegerOverflow=on
  Sum4 : Sum  Inputs=|++  SaturateOnIntegerOverflow=on
  Out1 : Outport  VectorParamsAs1DForOutWhenUnconnected=off
  wires:
  In1/1 -> Demux/1
  Demux/1 -> Sum3/2
  Constant1/1 -> Sum3/1
  Sum3/1 -> Product1/1
  Demux/2 -> Sum4/1
  Constant2/1 -> Sum4/2
  Sum4/1 -> Product1/2
  Product1/1 -> Out1/1

== system ap_12BAdapted/GlobalScope/DeHavilland Beaver Airframe/Aircraft Dynamics/Total Forces and Moments/Forces and Moments/Aero F&M/3x3 CrossProduct ==
  A : Inport
  B : Inport  Port=2
  "A " : InportShadow
  "B " : InportShadow  Port=2
  Subsystem : Subsystem
  Subsystem1 : Subsystem
  Sum : Sum  Inputs=+|-  SaturateOnIntegerOverflow=on  InputSameDT=on  OutDataTypeStr=Inherit: Same as first input
  C : Outport  VectorParamsAs1DForOutWhenUnconnected=off
  wires:
  "A "/1 -> Subsystem1/1(A)
  Subsystem/1(Out1) -> Sum/1
  B/1 -> Subsystem/2(B)
  Sum/1 -> C/1
  "B "/1 -> Subsystem1/2(B)
  Subsystem1/1(Out1) -> Sum/2
  A/1 -> Subsystem/1(A)

== system ap_12BAdapted/GlobalScope/DeHavilland Beaver Airframe/Aircraft Dynamics/Total Forces and Moments/Forces and Moments/Aero F&M/CG-CP Transformation ==
  Vb : Inport
  In : Inport  Port=2
  Terminator1 : Terminator
  Out : Outport  VectorParamsAs1DForOutWhenUnconnected=off
  wires:
  In/1 -> Out/1
  Vb/1 -> Terminator1/1

== system ap_12BAdapted/GlobalScope/DeHavilland Beaver Airframe/Aircraft Dynamics/Total Forces and Moments/Forces and Moments/Aero F&M/Force Transformation ==
  Vb : Inport
  In : Inport  Port=2
  Terminator1 : Terminator
  Out : Outport  VectorParamsAs1DForOutWhenUnconnected=off
  wires:
  In/1 -> Out/1
  Vb/1 -> Terminator1/1

== system ap_12BAdapted/GlobalScope/DeHavilland Beaver Airframe/Aircraft Dynamics/Total Forces and Moments/Forces and Moments/Aero F&M/Moment Transformation ==
  Vb : Inport
  In : Inport  Port=2
  Terminator1 : Terminator
  Out : Outport  VectorParamsAs1DForOutWhenUnconnected=off
  wires:
  In/1 -> Out/1
  Vb/1 -> Terminator1/1

== system ap_12BAdapted/GlobalScope/DeHavilland Beaver Airframe/Aircraft Dynamics/6DoF (Quaternion)/Calculate DCM & Euler Angles/Quaternions to Direction Cosine Matrix/Quaternion Normalize/Quaternion Modulus ==
  q : Inport  Unit=1
  Quaternion Norm : Subsystem  mask(Quaternion Norm){}
      mask help: shared_aeroblks:sharedaeroblkutil:blockQuaternionNormDesc
      mask init:
      | if license('test','aerospace_blockset')
      |     aerosharedicon('shared');
      | elseif license('test','powertrain_blockset')
      |     sharedautoicon('shared');
      | end
      mask Help: eval('if license(''test'',''aerospace_blockset'')aerosharedhelp;elseif license(''test'',''powertrain_blockset'')sharedautohelp;end')
  sqrt : Sqrt  AlgorithmType=Newton-Raphson  SaturateOnIntegerOverflow=on
  |q| : Outport  Unit=1  VectorParamsAs1DForOutWhenUnconnected=off
  wires:
  Quaternion Norm/1(norm(q)) -> sqrt/1
  q/1 -> Quaternion Norm/1(q)
  sqrt/1 -> |q|/1

== system ap_12BAdapted/GlobalScope/DeHavilland Beaver Airframe/Aircraft Dynamics/6DoF (Quaternion)/Calculate DCM & Euler Angles/Quaternions to Rotation Angles (ZYX)/Quaternion Normalize/Quaternion Modulus ==
  q : Inport
  Quaternion Norm : Subsystem
  sqrt : Sqrt  AlgorithmType=Newton-Raphson  SaturateOnIntegerOverflow=on
  |q| : Outport  VectorParamsAs1DForOutWhenUnconnected=off
  wires:
  Quaternion Norm/1(norm(q)) -> sqrt/1
  sqrt/1 -> |q|/1
  q/1 -> Quaternion Norm/1(q)

== system ap_12BAdapted/GlobalScope/DeHavilland Beaver Airframe/Aircraft Dynamics/Total Forces and Moments/Forces and Moments/Aero F&M/3x3 CrossProduct/Subsystem ==
  A : Inport
  B : Inport  Port=2
  Demux : Demux  Outputs=3
  Demux1 : Demux  Outputs=3
  Mux : Mux  Inputs=3
  i x j : Product  SaturateOnIntegerOverflow=on  InputSameDT=on  OutDataTypeStr=Inherit: Same as first input
  j x k : Product  SaturateOnIntegerOverflow=on  InputSameDT=on  OutDataTypeStr=Inherit: Same as first input
  k x i : Product  SaturateOnIntegerOverflow=on  InputSameDT=on  OutDataTypeStr=Inherit: Same as first input
  Out1 : Outport  VectorParamsAs1DForOutWhenUnconnected=off
  wires:
  Demux1/3 -> j x k/2
  Demux/2 -> j x k/1
  Demux/3 -> k x i/1
  Demux1/1 -> k x i/2
  Demux1/2 -> i x j/2
  Demux/1 -> i x j/1
  i x j/1 -> Mux/3
  k x i/1 -> Mux/2
  j x k/1 -> Mux/1
  B/1 -> Demux1/1
  A/1 -> Demux/1
  Mux/1 -> Out1/1

== system ap_12BAdapted/GlobalScope/DeHavilland Beaver Airframe/Aircraft Dynamics/Total Forces and Moments/Forces and Moments/Aero F&M/3x3 CrossProduct/Subsystem1 ==
  A : Inport
  B : Inport  Port=2
  Demux : Demux  Outputs=3
  Demux1 : Demux  Outputs=3
  Mux : Mux  Inputs=3
  i x k : Product  SaturateOnIntegerOverflow=on  InputSameDT=on  OutDataTypeStr=Inherit: Same as first input
  j x i : Product  SaturateOnIntegerOverflow=on  InputSameDT=on  OutDataTypeStr=Inherit: Same as first input
  k x j : Product  SaturateOnIntegerOverflow=on  InputSameDT=on  OutDataTypeStr=Inherit: Same as first input
  Out1 : Outport  VectorParamsAs1DForOutWhenUnconnected=off
  wires:
  j x i/1 -> Mux/3
  i x k/1 -> Mux/2
  k x j/1 -> Mux/1
  Mux/1 -> Out1/1
  Demux1/1 -> j x i/2
  Demux/2 -> j x i/1
  Demux1/3 -> i x k/2
  Demux/1 -> i x k/1
  Demux1/2 -> k x j/2
  Demux/3 -> k x j/1
  B/1 -> Demux1/1
  A/1 -> Demux/1

== system ap_12BAdapted/GlobalScope/DeHavilland Beaver Airframe/Aircraft Dynamics/6DoF (Quaternion)/Calculate DCM & Euler Angles/Quaternions to Direction Cosine Matrix/Quaternion Normalize/Quaternion Modulus/Quaternion Norm ==
  q : Inport  Unit=1
  Demux : Demux
  Product{,1..3} (4 alike) : Product
  Sum : Sum  Inputs=4
  norm(q) : Outport  Unit=1  VectorParamsAs1DForOutWhenUnconnected=off
  wires:
  Demux/4 -> Product3/1, Product3/2
  Demux/3 -> Product2/1, Product2/2
  Demux/2 -> Product1/1, Product1/2
  Demux/1 -> Product/1, Product/2
  Product3/1 -> Sum/4
  Product2/1 -> Sum/3
  Product1/1 -> Sum/2
  Product/1 -> Sum/1
  Sum/1 -> norm(q)/1
  q/1 -> Demux/1

== system ap_12BAdapted/GlobalScope/DeHavilland Beaver Airframe/Aircraft Dynamics/6DoF (Quaternion)/Calculate DCM & Euler Angles/Quaternions to Rotation Angles (ZYX)/Quaternion Normalize/Quaternion Modulus/Quaternion Norm ==
  q : Inport
  Demux : Demux
  Product{,1..3} (4 alike) : Product
  Sum : Sum  Inputs=4
  norm(q) : Outport  VectorParamsAs1DForOutWhenUnconnected=off
  wires:
  Demux/2 -> Product1/2, Product1/1
  q/1 -> Demux/1
  Sum/1 -> norm(q)/1
  Demux/1 -> Product/2, Product/1
  Product3/1 -> Sum/4
  Demux/3 -> Product2/2, Product2/1
  Product2/1 -> Sum/3
  Product/1 -> Sum/1
  Product1/1 -> Sum/2
  Demux/4 -> Product3/2, Product3/1
